simulink model "Parametrica"  (R2020b)
settings: Solver=VariableStepAuto  StartTime=0.0  StopTime=Smi.general.simulation_time  FixedStep=0.001  MaxStep=0.001  RelTol=1e-3  AbsTol=1e-3  EnableMultiTasking=on
undefined symbols (not defined in the file): Smi, X, Y, Z
libraries: sm_lib x754, nesl_utility x195, simulink x10, cstblocks x8, dspsrcs4 x6
(part 26 of 26)

== system Parametrica/MOVING CHASSIS/ACTUATOR RR/ACTUATOR IN//OUT/Random sine waves ==
  Clock : Clock
  Constant : Constant  Value=Smi.general.random_harshness
  Constant1 : Constant  Value=-100
  Divide : Product  Inputs=*/
  First Order Hold : FirstOrderHold  InitialOutput=-100  ErrorTolerance=30  AllowContinuousInput=on
  Gain : Gain  Gain=100
  Random Source : dspsrcs4/Random Source  SrcType=Uniform  NormMethod=Ziggurat  CltLength=12  MinVal=-Smi.general.random_amplitude*0.5  MaxVal=Smi.general.random_amplitude*0.5  MeanVal=0  VarVal=1  RepMode=Not repeatable  rawSeed=1  IsInherit=off  SampMode=Discrete  SampTime=0.05  SampFrame=1  DataType=Double  OutComplex=Real  OutputFrames=off
  Rate Transition : RateTransition  OutPortSampleTime=0
  Sum : Sum  Inputs=|+-
  Switch : Switch  Criteria=u2 ~= 0
  Varying Lowpass Filter : cstblocks/Linear Parameter Varying/Varying Lowpass Filter  N=5
  f : Outport
  wires:
  Constant/1 -> Varying Lowpass Filter/2
  Random Source/1 -> Rate Transition/1
  Divide/1 -> Gain/1
  Gain/1 -> Sum/2
  Varying Lowpass Filter/1 -> First Order Hold/1
  First Order Hold/1 -> Sum/1
  Clock/1 -> Divide/2, Switch/2, Divide/1
  Sum/1 -> Switch/1
  Constant1/1 -> Switch/3
  Switch/1 -> f/1
  Rate Transition/1 -> Varying Lowpass Filter/1

== system Parametrica/MOVING CHASSIS/BODY/FL HARDPOINTS/A forces sensing ==
  F : Inport
  Demux : Demux  Outputs=3
  To Workspace : ToWorkspace  VariableName=FL_A_Fx  SaveFormat=Timeseries  SampleTime=-1
  To Workspace1 : ToWorkspace  VariableName=FL_A_Fy  SaveFormat=Timeseries  SampleTime=-1
  To Workspace2 : ToWorkspace  VariableName=FL_A_Fz  SaveFormat=Timeseries  SampleTime=-1
  wires:
  Demux/1 -> To Workspace/1
  Demux/3 -> To Workspace2/1
  Demux/2 -> To Workspace1/1
  F/1 -> Demux/1

== system Parametrica/MOVING CHASSIS/BODY/FL HARDPOINTS/B forces sensing ==
  F : Inport
  Demux : Demux  Outputs=3
  To Workspace : ToWorkspace  VariableName=FL_B_Fx  SaveFormat=Timeseries  SampleTime=-1
  To Workspace1 : ToWorkspace  VariableName=FL_B_Fy  SaveFormat=Timeseries  SampleTime=-1
  To Workspace2 : ToWorkspace  VariableName=FL_B_Fz  SaveFormat=Timeseries  SampleTime=-1
  wires:
  Demux/1 -> To Workspace/1
  Demux/3 -> To Workspace2/1
  Demux/2 -> To Workspace1/1
  F/1 -> Demux/1

== system Parametrica/MOVING CHASSIS/BODY/FL HARDPOINTS/C forces sensing ==
  F : Inport
  Demux : Demux  Outputs=3
  To Workspace : ToWorkspace  VariableName=FL_C_Fx  SaveFormat=Timeseries  SampleTime=-1
  To Workspace1 : ToWorkspace  VariableName=FL_C_Fy  SaveFormat=Timeseries  SampleTime=-1
  To Workspace2 : ToWorkspace  VariableName=FL_C_Fz  SaveFormat=Timeseries  SampleTime=-1
  wires:
  Demux/1 -> To Workspace/1
  Demux/3 -> To Workspace2/1
  Demux/2 -> To Workspace1/1
  F/1 -> Demux/1

== system Parametrica/MOVING CHASSIS/BODY/FL HARDPOINTS/D forces sensing ==
  F : Inport
  Demux : Demux  Outputs=3
  To Workspace : ToWorkspace  VariableName=FL_D_Fx  SaveFormat=Timeseries  SampleTime=-1
  To Workspace1 : ToWorkspace  VariableName=FL_D_Fy  SaveFormat=Timeseries  SampleTime=-1
  To Workspace2 : ToWorkspace  VariableName=FL_D_Fz  SaveFormat=Timeseries  SampleTime=-1
  wires:
  Demux/1 -> To Workspace/1
  Demux/3 -> To Workspace2/1
  Demux/2 -> To Workspace1/1
  F/1 -> Demux/1

== system Parametrica/MOVING CHASSIS/BODY/FL HARDPOINTS/crank forces sensing ==
  F : Inport
  Demux : Demux  Outputs=3
  To Workspace : ToWorkspace  VariableName=FL_CRANK_Fx  SaveFormat=Timeseries  SampleTime=-1
  To Workspace1 : ToWorkspace  VariableName=FL_CRANK_Fy  SaveFormat=Timeseries  SampleTime=-1
  To Workspace2 : ToWorkspace  VariableName=FL_CRANK_Fz  SaveFormat=Timeseries  SampleTime=-1
  wires:
  Demux/1 -> To Workspace/1
  Demux/3 -> To Workspace2/1
  Demux/2 -> To Workspace1/1
  F/1 -> Demux/1

== system Parametrica/MOVING CHASSIS/BODY/FL HARDPOINTS/damper forces sensing ==
  F : Inport
  Demux : Demux  Outputs=3
  To Workspace : ToWorkspace  VariableName=FL_AMMO_Fx  SaveFormat=Timeseries  SampleTime=-1
  To Workspace1 : ToWorkspace  VariableName=FL_AMMO_Fy  SaveFormat=Timeseries  SampleTime=-1
  To Workspace2 : ToWorkspace  VariableName=FL_AMMO_Fz  SaveFormat=Timeseries  SampleTime=-1
  wires:
  Demux/1 -> To Workspace/1
  Demux/3 -> To Workspace2/1
  Demux/2 -> To Workspace1/1
  F/1 -> Demux/1

== system Parametrica/MOVING CHASSIS/BODY/FR HARDPOINTS/A forces sensing ==
  F : Inport
  Demux : Demux  Outputs=3
  To Workspace : ToWorkspace  VariableName=FR_A_Fx  SaveFormat=Timeseries  SampleTime=-1
  To Workspace1 : ToWorkspace  VariableName=FR_A_Fy  SaveFormat=Timeseries  SampleTime=-1
  To Workspace2 : ToWorkspace  VariableName=FR_A_Fz  SaveFormat=Timeseries  SampleTime=-1
  wires:
  Demux/1 -> To Workspace/1
  Demux/3 -> To Workspace2/1
  Demux/2 -> To Workspace1/1
  F/1 -> Demux/1

== system Parametrica/MOVING CHASSIS/BODY/FR HARDPOINTS/B forces sensing ==
  F : Inport
  Demux : Demux  Outputs=3
  To Workspace : ToWorkspace  VariableName=FR_B_Fx  SaveFormat=Timeseries  SampleTime=-1
  To Workspace1 : ToWorkspace  VariableName=FR_B_Fy  SaveFormat=Timeseries  SampleTime=-1
  To Workspace2 : ToWorkspace  VariableName=FR_B_Fz  SaveFormat=Timeseries  SampleTime=-1
  wires:
  Demux/1 -> To Workspace/1
  Demux/3 -> To Workspace2/1
  Demux/2 -> To Workspace1/1
  F/1 -> Demux/1

== system Parametrica/MOVING CHASSIS/BODY/FR HARDPOINTS/C forces sensing ==
  F : Inport
  Demux : Demux  Outputs=3
  To Workspace : ToWorkspace  VariableName=FR_C_Fx  SaveFormat=Timeseries  SampleTime=-1
  To Workspace1 : ToWorkspace  VariableName=FR_C_Fy  SaveFormat=Timeseries  SampleTime=-1
  To Workspace2 : ToWorkspace  VariableName=FR_C_Fz  SaveFormat=Timeseries  SampleTime=-1
  wires:
  Demux/1 -> To Workspace/1
  Demux/3 -> To Workspace2/1
  Demux/2 -> To Workspace1/1
  F/1 -> Demux/1

== system Parametrica/MOVING CHASSIS/BODY/FR HARDPOINTS/D forces sensing ==
  F : Inport
  Demux : Demux  Outputs=3
  To Workspace : ToWorkspace  VariableName=FR_D_Fx  SaveFormat=Timeseries  SampleTime=-1
  To Workspace1 : ToWorkspace  VariableName=FR_D_Fy  SaveFormat=Timeseries  SampleTime=-1
  To Workspace2 : ToWorkspace  VariableName=FR_D_Fz  SaveFormat=Timeseries  SampleTime=-1
  wires:
  Demux/1 -> To Workspace/1
  Demux/3 -> To Workspace2/1
  Demux/2 -> To Workspace1/1
  F/1 -> Demux/1

== system Parametrica/MOVING CHASSIS/BODY/FR HARDPOINTS/crank forces sensing ==
  F : Inport
  Demux : Demux  Outputs=3
  To Workspace : ToWorkspace  VariableName=FR_CRANK_Fx  SaveFormat=Timeseries  SampleTime=-1
  To Workspace1 : ToWorkspace  VariableName=FR_CRANK_Fy  SaveFormat=Timeseries  SampleTime=-1
  To Workspace2 : ToWorkspace  VariableName=FR_CRANK_Fz  SaveFormat=Timeseries  SampleTime=-1
  wires:
  Demux/1 -> To Workspace/1
  Demux/3 -> To Workspace2/1
  Demux/2 -> To Workspace1/1
  F/1 -> Demux/1

== system Parametrica/MOVING CHASSIS/BODY/FR HARDPOINTS/damper forces sensing ==
  F : Inport
  Demux : Demux  Outputs=3
  To Workspace : ToWorkspace  VariableName=FR_AMMO_Fx  SaveFormat=Timeseries  SampleTime=-1
  To Workspace1 : ToWorkspace  VariableName=FR_AMMO_Fy  SaveFormat=Timeseries  SampleTime=-1
  To Workspace2 : ToWorkspace  VariableName=FR_AMMO_Fz  SaveFormat=Timeseries  SampleTime=-1
  wires:
  Demux/1 -> To Workspace/1
  Demux/3 -> To Workspace2/1
  Demux/2 -> To Workspace1/1
  F/1 -> Demux/1

== system Parametrica/MOVING CHASSIS/BODY/RL HARDPOINTS/A forces sensing ==
  F : Inport
  Demux : Demux  Outputs=3
  To Workspace : ToWorkspace  VariableName=RL_A_Fx  SaveFormat=Timeseries  SampleTime=-1
  To Workspace1 : ToWorkspace  VariableName=RL_A_Fy  SaveFormat=Timeseries  SampleTime=-1
  To Workspace2 : ToWorkspace  VariableName=RL_A_Fz  SaveFormat=Timeseries  SampleTime=-1
  wires:
  Demux/1 -> To Workspace/1
  Demux/3 -> To Workspace2/1
  Demux/2 -> To Workspace1/1
  F/1 -> Demux/1

== system Parametrica/MOVING CHASSIS/BODY/RL HARDPOINTS/B forces sensing ==
  F : Inport
  Demux : Demux  Outputs=3
  To Workspace : ToWorkspace  VariableName=RL_B_Fx  SaveFormat=Timeseries  SampleTime=-1
  To Workspace1 : ToWorkspace  VariableName=RL_B_Fy  SaveFormat=Timeseries  SampleTime=-1
  To Workspace2 : ToWorkspace  VariableName=RL_B_Fz  SaveFormat=Timeseries  SampleTime=-1
  wires:
  Demux/1 -> To Workspace/1
  Demux/3 -> To Workspace2/1
  Demux/2 -> To Workspace1/1
  F/1 -> Demux/1

== system Parametrica/MOVING CHASSIS/BODY/RL HARDPOINTS/C forces sensing ==
  F : Inport
  Demux : Demux  Outputs=3
  To Workspace : ToWorkspace  VariableName=RL_C_Fx  SaveFormat=Timeseries  SampleTime=-1
  To Workspace1 : ToWorkspace  VariableName=RL_C_Fy  SaveFormat=Timeseries  SampleTime=-1
  To Workspace2 : ToWorkspace  VariableName=RL_C_Fz  SaveFormat=Timeseries  SampleTime=-1
  wires:
  Demux/1 -> To Workspace/1
  Demux/3 -> To Workspace2/1
  Demux/2 -> To Workspace1/1
  F/1 -> Demux/1

== system Parametrica/MOVING CHASSIS/BODY/RL HARDPOINTS/D forces sensing ==
  F : Inport
  Demux : Demux  Outputs=3
  To Workspace : ToWorkspace  VariableName=RL_D_Fx  SaveFormat=Timeseries  SampleTime=-1
  To Workspace1 : ToWorkspace  VariableName=RL_D_Fy  SaveFormat=Timeseries  SampleTime=-1
  To Workspace2 : ToWorkspace  VariableName=RL_D_Fz  SaveFormat=Timeseries  SampleTime=-1
  wires:
  Demux/1 -> To Workspace/1
  Demux/3 -> To Workspace2/1
  Demux/2 -> To Workspace1/1
  F/1 -> Demux/1

== system Parametrica/MOVING CHASSIS/BODY/RL HARDPOINTS/crank forces sensing ==
  F : Inport
  Demux : Demux  Outputs=3
  To Workspace : ToWorkspace  VariableName=RL_CRANK_Fx  SaveFormat=Timeseries  SampleTime=-1
  To Workspace1 : ToWorkspace  VariableName=RL_CRANK_Fy  SaveFormat=Timeseries  SampleTime=-1
  To Workspace2 : ToWorkspace  VariableName=RL_CRANK_Fz  SaveFormat=Timeseries  SampleTime=-1
  wires:
  Demux/1 -> To Workspace/1
  Demux/3 -> To Workspace2/1
  Demux/2 -> To Workspace1/1
  F/1 -> Demux/1

== system Parametrica/MOVING CHASSIS/BODY/RL HARDPOINTS/damper forces sensing ==
  F : Inport
  Demux : Demux  Outputs=3
  To Workspace : ToWorkspace  VariableName=RL_AMMO_Fx  SaveFormat=Timeseries  SampleTime=-1
  To Workspace1 : ToWorkspace  VariableName=RL_AMMO_Fy  SaveFormat=Timeseries  SampleTime=-1
  To Workspace2 : ToWorkspace  VariableName=RL_AMMO_Fz  SaveFormat=Timeseries  SampleTime=-1
  wires:
  Demux/1 -> To Workspace/1
  Demux/3 -> To Workspace2/1
  Demux/2 -> To Workspace1/1
  F/1 -> Demux/1

== system Parametrica/MOVING CHASSIS/BODY/RR HARDPOINTS/A forces sensing ==
  F : Inport
  Demux : Demux  Outputs=3
  To Workspace : ToWorkspace  VariableName=RR_A_Fx  SaveFormat=Timeseries  SampleTime=-1
  To Workspace1 : ToWorkspace  VariableName=RR_A_Fy  SaveFormat=Timeseries  SampleTime=-1
  To Workspace2 : ToWorkspace  VariableName=RR_A_Fz  SaveFormat=Timeseries  SampleTime=-1
  wires:
  Demux/1 -> To Workspace/1
  Demux/3 -> To Workspace2/1
  Demux/2 -> To Workspace1/1
  F/1 -> Demux/1

== system Parametrica/MOVING CHASSIS/BODY/RR HARDPOINTS/B forces sensing ==
  F : Inport
  Demux : Demux  Outputs=3
  To Workspace : ToWorkspace  VariableName=RR_B_Fx  SaveFormat=Timeseries  SampleTime=-1
  To Workspace1 : ToWorkspace  VariableName=RR_B_Fy  SaveFormat=Timeseries  SampleTime=-1
  To Workspace2 : ToWorkspace  VariableName=RR_B_Fz  SaveFormat=Timeseries  SampleTime=-1
  wires:
  Demux/1 -> To Workspace/1
  Demux/3 -> To Workspace2/1
  Demux/2 -> To Workspace1/1
  F/1 -> Demux/1

== system Parametrica/MOVING CHASSIS/BODY/RR HARDPOINTS/C forces sensing ==
  F : Inport
  Demux : Demux  Outputs=3
  To Workspace : ToWorkspace  VariableName=RR_C_Fx  SaveFormat=Timeseries  SampleTime=-1
  To Workspace1 : ToWorkspace  VariableName=RR_C_Fy  SaveFormat=Timeseries  SampleTime=-1
  To Workspace2 : ToWorkspace  VariableName=RR_C_Fz  SaveFormat=Timeseries  SampleTime=-1
  wires:
  Demux/1 -> To Workspace/1
  Demux/3 -> To Workspace2/1
  Demux/2 -> To Workspace1/1
  F/1 -> Demux/1

== system Parametrica/MOVING CHASSIS/BODY/RR HARDPOINTS/D forces sensing ==
  F : Inport
  Demux : Demux  Outputs=3
  To Workspace : ToWorkspace  VariableName=RR_D_Fx  SaveFormat=Timeseries  SampleTime=-1
  To Workspace1 : ToWorkspace  VariableName=RR_D_Fy  SaveFormat=Timeseries  SampleTime=-1
  To Workspace2 : ToWorkspace  VariableName=RR_D_Fz  SaveFormat=Timeseries  SampleTime=-1
  wires:
  Demux/1 -> To Workspace/1
  Demux/3 -> To Workspace2/1
  Demux/2 -> To Workspace1/1
  F/1 -> Demux/1

== system Parametrica/MOVING CHASSIS/BODY/RR HARDPOINTS/crank forces sensing ==
  F : Inport
  Demux : Demux  Outputs=3
  To Workspace : ToWorkspace  VariableName=RR_CRANK_Fx  SaveFormat=Timeseries  SampleTime=-1
  To Workspace1 : ToWorkspace  VariableName=RR_CRANK_Fy  SaveFormat=Timeseries  SampleTime=-1
  To Workspace2 : ToWorkspace  VariableName=RR_CRANK_Fz  SaveFormat=Timeseries  SampleTime=-1
  wires:
  Demux/1 -> To Workspace/1
  Demux/3 -> To Workspace2/1
  Demux/2 -> To Workspace1/1
  F/1 -> Demux/1

== system Parametrica/MOVING CHASSIS/BODY/RR HARDPOINTS/damper forces sensing ==
  F : Inport
  Demux : Demux  Outputs=3
  To Workspace : ToWorkspace  VariableName=RR_AMMO_Fx  SaveFormat=Timeseries  SampleTime=-1
  To Workspace1 : ToWorkspace  VariableName=RR_AMMO_Fy  SaveFormat=Timeseries  SampleTime=-1
  To Workspace2 : ToWorkspace  VariableName=RR_AMMO_Fz  SaveFormat=Timeseries  SampleTime=-1
  wires:
  Demux/1 -> To Workspace/1
  Demux/3 -> To Workspace2/1
  Demux/2 -> To Workspace1/1
  F/1 -> Demux/1
